simulink model "SP_Dynamic_17Okt_ExergyFlow"  (R2019b)
settings: Solver=FixedStepAuto  StartTime=0.0  StopTime=0  FixedStep=1/3600  RelTol=1e-3
model workspace (MAT data in the model file):
  AD : Simulink.Parameter (value not decoded)
  AG : Simulink.Parameter (value not decoded)
  AH : Simulink.Parameter (value not decoded)
  AV : Simulink.Parameter (value not decoded)
  AVP : Simulink.Parameter (value not decoded)
  BCHL : Simulink.Parameter (value not decoded)
  BCHV : Simulink.Parameter (value not decoded)
  BD : Simulink.Parameter (value not decoded)
  BG : Simulink.Parameter (value not decoded)
  BH : Simulink.Parameter (value not decoded)
  BVP : Simulink.Parameter (value not decoded)
  CD : Simulink.Parameter (value not decoded)
  CG : Simulink.Parameter (value not decoded)
  CH : Simulink.Parameter (value not decoded)
  CVP : Simulink.Parameter (value not decoded)
  XMW : Simulink.Parameter (value not decoded)
symbols that are objects in the model workspace (value not decoded): AD, AG, AH, AV, AVP, BD, BG, BH, BVP, CD, CG, CH, CVP, XMW
undefined symbols (not defined in the file or in its folder): magnitude, SETPT, XMEAS, XMV
libraries: mylib x165, dspindex x17
(part 6 of 10)

== system SP_Dynamic_17Okt_ExergyFlow/Reactor/Holdup of Components in Reactor/YP(3) ==
  FCM(3,7) : Inport
  CRXR(3) : Inport  Port=2
  FCM(3,8) : Inport  Port=3
  " " : Sum  Inputs=+-+
  Bus Selector : BusSelector  OutputSignals=CRXR(3)
  Bus Selector1 : BusSelector  OutputSignals=FCM(3;8)
  Bus Selector2 : BusSelector  OutputSignals=FCM(3;7)
  YP(3) : Integrator  InitialConditionSource=external
  "YY(3) " : Constant  Value=7.5700579737
  YY(3) : Outport  VectorParamsAs1DForOutWhenUnconnected=off
  wires:
  "YY(3) "/1 -> YP(3)/2
  CRXR(3)/1 -> Bus Selector/1
  FCM(3,8)/1 -> Bus Selector1/1
  FCM(3,7)/1 -> Bus Selector2/1
  " "/1 -> YP(3)/1
  YP(3)/1 -> YY(3)/1
  Bus Selector/1 -> " "/3  "<CRXR(3)>"
  Bus Selector1/1 -> " "/2  "<FCM(3;8)>"
  Bus Selector2/1 -> " "/1  "<FCM(3;7)>"

== system SP_Dynamic_17Okt_ExergyFlow/Reactor/Holdup of Components in Reactor/YP(4) ==
  FCM(4,7) : Inport
  CRXR(4) : Inport  Port=2
  FCM(4,8) : Inport  Port=3
  " " : Sum  Inputs=+-+
  Bus Selector : BusSelector  OutputSignals=CRXR(4)
  Bus Selector1 : BusSelector  OutputSignals=FCM(4;8)
  Bus Selector2 : BusSelector  OutputSignals=FCM(4;7)
  YP(4) : Integrator  InitialConditionSource=external
  YY(4) : Constant  Value=0.4230042431
  "YY(4) " : Outport  VectorParamsAs1DForOutWhenUnconnected=off
  wires:
  YY(4)/1 -> YP(4)/2
  CRXR(4)/1 -> Bus Selector/1
  FCM(4,8)/1 -> Bus Selector1/1
  FCM(4,7)/1 -> Bus Selector2/1
  " "/1 -> YP(4)/1
  YP(4)/1 -> "YY(4) "/1
  Bus Selector/1 -> " "/3  "<CRXR(4)>"
  Bus Selector1/1 -> " "/2  "<FCM(4;8)>"
  Bus Selector2/1 -> " "/1  "<FCM(4;7)>"

== system SP_Dynamic_17Okt_ExergyFlow/Reactor/Holdup of Components in Reactor/YP(5) ==
  FCM(5,7) : Inport
  CRXR(5) : Inport  Port=2
  FCM(5,8) : Inport  Port=3
  " " : Sum  Inputs=+-+
  Bus Selector : BusSelector  OutputSignals=CRXR(5)
  Bus Selector1 : BusSelector  OutputSignals=FCM(5;8)
  Bus Selector2 : BusSelector  OutputSignals=FCM(5;7)
  YP(5) : Integrator  InitialConditionSource=external
  YY(5) : Constant  Value=24.15513437
  "YY(5) " : Outport  VectorParamsAs1DForOutWhenUnconnected=off
  wires:
  YY(5)/1 -> YP(5)/2
  CRXR(5)/1 -> Bus Selector/1
  FCM(5,8)/1 -> Bus Selector1/1
  FCM(5,7)/1 -> Bus Selector2/1
  " "/1 -> YP(5)/1
  YP(5)/1 -> "YY(5) "/1
  Bus Selector/1 -> " "/3  "<CRXR(5)>"
  Bus Selector1/1 -> " "/2  "<FCM(5;8)>"
  Bus Selector2/1 -> " "/1  "<FCM(5;7)>"

== system SP_Dynamic_17Okt_ExergyFlow/Reactor/Holdup of Components in Reactor/YP(6) ==
  FCM(6,7) : Inport
  CRXR(6) : Inport  Port=2
  FCM(6,8) : Inport  Port=3
  " " : Sum  Inputs=+-+
  Bus Selector : BusSelector  OutputSignals=CRXR(6)
  Bus Selector1 : BusSelector  OutputSignals=FCM(6;8)
  Bus Selector2 : BusSelector  OutputSignals=FCM(6;7)
  YP(6) : Integrator  InitialConditionSource=external
  YY(6) : Constant  Value=2.942597645
  "YY(6) " : Outport  VectorParamsAs1DForOutWhenUnconnected=off
  wires:
  YY(6)/1 -> YP(6)/2
  CRXR(6)/1 -> Bus Selector/1
  FCM(6,8)/1 -> Bus Selector1/1
  FCM(6,7)/1 -> Bus Selector2/1
  " "/1 -> YP(6)/1
  YP(6)/1 -> "YY(6) "/1
  Bus Selector/1 -> " "/3  "<CRXR(6)>"
  Bus Selector1/1 -> " "/2  "<FCM(6;8)>"
  Bus Selector2/1 -> " "/1  "<FCM(6;7)>"

== system SP_Dynamic_17Okt_ExergyFlow/Reactor/Holdup of Components in Reactor/YP(7) ==
  FCM(7,7) : Inport
  CRXR(7) : Inport  Port=2
  FCM(7,8) : Inport  Port=3
  " " : Sum  Inputs=+-+
  Bus Selector : BusSelector  OutputSignals=CRXR(7)
  Bus Selector1 : BusSelector  OutputSignals=FCM(7;8)
  Bus Selector2 : BusSelector  OutputSignals=FCM(7;7)
  YP(7) : Integrator  InitialConditionSource=external
  YY(7) : Constant  Value=154.3770655
  "YY(7) " : Outport  VectorParamsAs1DForOutWhenUnconnected=off
  wires:
  YY(7)/1 -> YP(7)/2
  CRXR(7)/1 -> Bus Selector/1
  FCM(7,8)/1 -> Bus Selector1/1
  FCM(7,7)/1 -> Bus Selector2/1
  " "/1 -> YP(7)/1
  YP(7)/1 -> "YY(7) "/1
  Bus Selector/1 -> " "/3  "<CRXR(7)>"
  Bus Selector1/1 -> " "/2  "<FCM(7;8)>"
  Bus Selector2/1 -> " "/1  "<FCM(7;7)>"

== system SP_Dynamic_17Okt_ExergyFlow/Reactor/Holdup of Components in Reactor/YP(8) ==
  FCM(8,7) : Inport
  CRXR(8) : Inport  Port=2
  FCM(8,8) : Inport  Port=3
  " " : Sum  Inputs=+-+
  Bus Selector : BusSelector  OutputSignals=CRXR(8)
  Bus Selector1 : BusSelector  OutputSignals=FCM(8;8)
  Bus Selector2 : BusSelector  OutputSignals=FCM(8;7)
  YP(8) : Integrator  InitialConditionSource=external
  YY(8) : Constant  Value=159.1865960
  "YY(8) " : Outport  VectorParamsAs1DForOutWhenUnconnected=off
  wires:
  YY(8)/1 -> YP(8)/2
  CRXR(8)/1 -> Bus Selector/1
  FCM(8,8)/1 -> Bus Selector1/1
  FCM(8,7)/1 -> Bus Selector2/1
  " "/1 -> YP(8)/1
  YP(8)/1 -> "YY(8) "/1
  Bus Selector/1 -> " "/3  "<CRXR(8)>"
  Bus Selector1/1 -> " "/2  "<FCM(8;8)>"
  Bus Selector2/1 -> " "/1  "<FCM(8;7)>"

== system SP_Dynamic_17Okt_ExergyFlow/Reactor/Pressure of Reactor/Subsystem ==
  TKR : Inport
  VVR : Inport  Port=2
  UCVR : Inport  Port=3
  Bus Selector : BusSelector  OutputSignals=UCVR(1),UCVR(2),UCVR(3)
  PPR(1) Partial pressure of Component A mmHg : Product  Inputs=***/
  PPR(2) Partial pressure of Component B mmHg : Product  Inputs=***/
  PPR(3) Partial pressure of Component C mmHg : Product  Inputs=***/
  RG Universal Gas Constant ft³·mmHg/K·lb-mol : Constant  Value=998.9
  PPR(1) : Outport  VectorParamsAs1DForOutWhenUnconnected=off
  PPR(2) : Outport  Port=2  VectorParamsAs1DForOutWhenUnconnected=off
  PPR(3) : Outport  Port=3  VectorParamsAs1DForOutWhenUnconnected=off
  wires:
  Bus Selector/2 -> PPR(2) Partial pressure of Component B mmHg/1  "<UCVR(2)>"
  TKR/1 -> PPR(3) Partial pressure of Component C mmHg/3, PPR(2) Partial pressure of Component B mmHg/3, PPR(1) Partial pressure of Component A mmHg/3
  VVR/1 -> PPR(3) Partial pressure of Component C mmHg/4, PPR(2) Partial pressure of Component B mmHg/4, PPR(1) Partial pressure of Component A mmHg/4
  RG Universal Gas Constant ft³·mmHg/K·lb-mol/1 -> PPR(3) Partial pressure of Component C mmHg/2, PPR(1) Partial pressure of Component A mmHg/2, PPR(2) Partial pressure of Component B mmHg/2
  PPR(2) Partial pressure of Component B mmHg/1 -> PPR(2)/1  "PPR(2)"
  Bus Selector/1 -> PPR(1) Partial pressure of Component A mmHg/1  "<UCVR(1)>"
  Bus Selector/3 -> PPR(3) Partial pressure of Component C mmHg/1  "<UCVR(3)>"
  PPR(1) Partial pressure of Component A mmHg/1 -> PPR(1)/1  "PPR(1)"
  PPR(3) Partial pressure of Component C mmHg/1 -> PPR(3)/1  "PPR(3)"
  UCVR/1 -> Bus Selector/1

== system SP_Dynamic_17Okt_ExergyFlow/Reactor/Pressure of Reactor/VPR Vapour Pressure mmHg ==
  TCR : Inport
  AVP(I) Antoine Coefficient A ln(mmHg) : Constant  Value=AVP
  Add : Sum
  Add1 : Sum
  BVP(I) Antoine Coefficient B ln(mmHg)·°C : Constant  Value=BVP
  CVP(I) Antoine Coefficient C °C : Constant  Value=CVP
  Divide : Product  Inputs=*/
  Math Function : Math  SaturateOnIntegerOverflow=on
  VPR : Outport  VectorParamsAs1DForOutWhenUnconnected=off
  wires:
  BVP(I) Antoine Coefficient B ln(mmHg)·°C/1 -> Divide/1
  CVP(I) Antoine Coefficient C °C/1 -> Add/1
  AVP(I) Antoine Coefficient A ln(mmHg)/1 -> Add1/1
  Add/1 -> Divide/2
  Divide/1 -> Add1/2
  Add1/1 -> Math Function/1
  Math Function/1 -> VPR/1
  TCR/1 -> Add/2

== system SP_Dynamic_17Okt_ExergyFlow/Reactor/Reaction Rates/Component reaction rate lb-mol//h ==
  RR : Inport
  Bus Creator : BusCreator  Inputs=7
  Subsystem : Subsystem
  Subsystem1 : Subsystem
  Subsystem2 : Subsystem
  Subsystem3 : Subsystem
  Subsystem4 : Subsystem
  Subsystem5 : Subsystem
  Subsystem6 : Subsystem
  CRXR : Outport  VectorParamsAs1DForOutWhenUnconnected=off
  wires:
  RR/1 -> Subsystem4/1(RR), Subsystem6/1(RR), Subsystem5/1(RR), Subsystem3/1(RR), Subsystem1/1(RR), Subsystem/1(RR), Subsystem2/1(RR)
  Bus Creator/1 -> CRXR/1
  Subsystem/1(CRXR(1)) -> Bus Creator/1
  Subsystem1/1(CRXR(3)) -> Bus Creator/2
  Subsystem2/1(CRXR(4)) -> Bus Creator/3
  Subsystem3/1(CRXR(5)) -> Bus Creator/4
  Subsystem4/1(CRXR(6)) -> Bus Creator/5
  Subsystem5/1(CRXR(7)) -> Bus Creator/6
  Subsystem6/1(CRXR(8)) -> Bus Creator/7

== system SP_Dynamic_17Okt_ExergyFlow/Reactor/Reaction Rates/Reaction Heat MBtu//h ==
  RR : Inport
  Bus Selector : BusSelector  OutputSignals=RR(1),RR(2)
  HTR(1) Heat of Reaction 1 MBtu/lb-mol : Constant  Value=0.06899381054
  HTR(2) Heat of reaction 2 MBtu/lb-mol : Constant  Value=0.05
  Product : Product
  Product1 : Product
  RH Total reaction heat MBtu/h : Sum
  RH : Outport  VectorParamsAs1DForOutWhenUnconnected=off
  wires:
  HTR(2) Heat of reaction 2 MBtu/lb-mol/1 -> Product1/2
  Product/1 -> RH Total reaction heat MBtu/h/1
  Product1/1 -> RH Total reaction heat MBtu/h/2
  HTR(1) Heat of Reaction 1 MBtu/lb-mol/1 -> Product/2
  RH Total reaction heat MBtu/h/1 -> RH/1
  RR/1 -> Bus Selector/1
  Bus Selector/1 -> Product/1  "<RR(1)>"
  Bus Selector/2 -> Product1/1  "<RR(2)>"

== system SP_Dynamic_17Okt_ExergyFlow/Reactor/Reaction Rates/Reaction rates lb-mol//h ==
  TKR : Inport
  PPR : Inport  Port=2
  VVR : Inport  Port=3
  " Reaction rate of reaction 4 lb-mol/ft3·h    " : Subsystem
  Bus Creator : BusCreator  Inputs=4
  Product{,1..3} (4 alike) : Product
  Reaction rate of reaction 1 lb-mol/ft3·h : Subsystem
  Reaction rate of reaction 2 lb-mol/ft3·h : Subsystem
  "Reaction rate of reaction 3 lb-mol/ft3·h  " : Subsystem
  RR : Outport  VectorParamsAs1DForOutWhenUnconnected=off
  wires:
  TKR/1 -> Reaction rate of reaction 1 lb-mol/ft3·h/2(TKR), " Reaction rate of reaction 4 lb-mol/ft3·h    "/2(TKR), "Reaction rate of reaction 3 lb-mol/ft3·h  "/2(TKR), Reaction rate of reaction 2 lb-mol/ft3·h/2(TKR)
  PPR/1 -> Reaction rate of reaction 1 lb-mol/ft3·h/1(PPR), " Reaction rate of reaction 4 lb-mol/ft3·h    "/1(PPR), "Reaction rate of reaction 3 lb-mol/ft3·h  "/1(PPR), Reaction rate of reaction 2 lb-mol/ft3·h/1(PPR)
  Bus Creator/1 -> RR/1
  Reaction rate of reaction 1 lb-mol/ft3·h/1(RR(1)) -> Product/1  "RR(1)"
  VVR/1 -> Product/2, Product3/2, Product2/2, Product1/2
  Product/1 -> Bus Creator/1  "RR(1)"
  Reaction rate of reaction 2 lb-mol/ft3·h/1(RR(2)) -> Product1/1  "RR(2)"
  Product1/1 -> Bus Creator/2  "RR(2)"
  "Reaction rate of reaction 3 lb-mol/ft3·h  "/1(RR(3)) -> Product2/1  "RR(3)"
  Product2/1 -> Bus Creator/3  "RR(3)"
  " Reaction rate of reaction 4 lb-mol/ft3·h    "/1(RR(4)) -> Product3/1  "RR(4)"
  Product3/1 -> Bus Creator/4  "RR(4)"

== system SP_Dynamic_17Okt_ExergyFlow/Reactor/Reactor Heat exchanger/Position of Valve 10 % ==
  Bus Selector : BusSelector  OutputSignals=XMV(10)
  Bus Selector1 : BusSelector  OutputSignals=IDV(14)
  Control valve : mylib/Control valve  SystemSampleTime=-1  Latency=0  AutoFrameSizeCalculation=off
  Divide : Product  Inputs=*/
  Subtract : Sum  Inputs=+-
  VTAU(10) : Constant  Value=5/3600
  YP(48) : Integrator  InitialConditionSource=external
  YY(48) : Constant  Value=41.10581288
  "YY(48) " : Outport  PortDimensions=1  VectorParamsAs1DForOutWhenUnconnected=off
  wires:
  YP(48)/1 -> Subtract/2, "YY(48) "/1  "VPOS(10)"
  Subtract/1 -> Divide/1
  Control valve/1 -> Subtract/1
  VTAU(10)/1 -> Divide/2
  Divide/1 -> YP(48)/1
  YY(48)/1 -> YP(48)/2
  [XMV] -> Bus Selector/1
  Bus Selector/1 -> Control valve/1  "<XMV(10)>"
  [IDV] -> Bus Selector1/1
  Bus Selector1/1 -> Control valve/2  "<IDV(14)>"

== system SP_Dynamic_17Okt_ExergyFlow/Reactor/Reactor Heat exchanger/Position of Valve 12 % ==
  Bus Selector : BusSelector  OutputSignals=XMV(12)
  Control valve : Subsystem
  Divide : Product  Inputs=*/
  Subtract : Sum  Inputs=+-
  VTAU(12) : Constant  Value=5/3600
  YP(50) : Integrator  InitialConditionSource=external
  YY(50) : Constant  Value=50
  "YY(50) " : Outport  PortDimensions=1  VectorParamsAs1DForOutWhenUnconnected=off
  wires:
  YP(50)/1 -> Subtract/2, "YY(50) "/1  "VPOS(12)"
  Subtract/1 -> Divide/1
  Control valve/1(VCV(12)) -> Subtract/1
  VTAU(12)/1 -> Divide/2
  Divide/1 -> YP(50)/1
  YY(50)/1 -> YP(50)/2
  [XMV] -> Bus Selector/1
  Bus Selector/1 -> Control valve/1(XMV(12))  "<XMV(12)>"

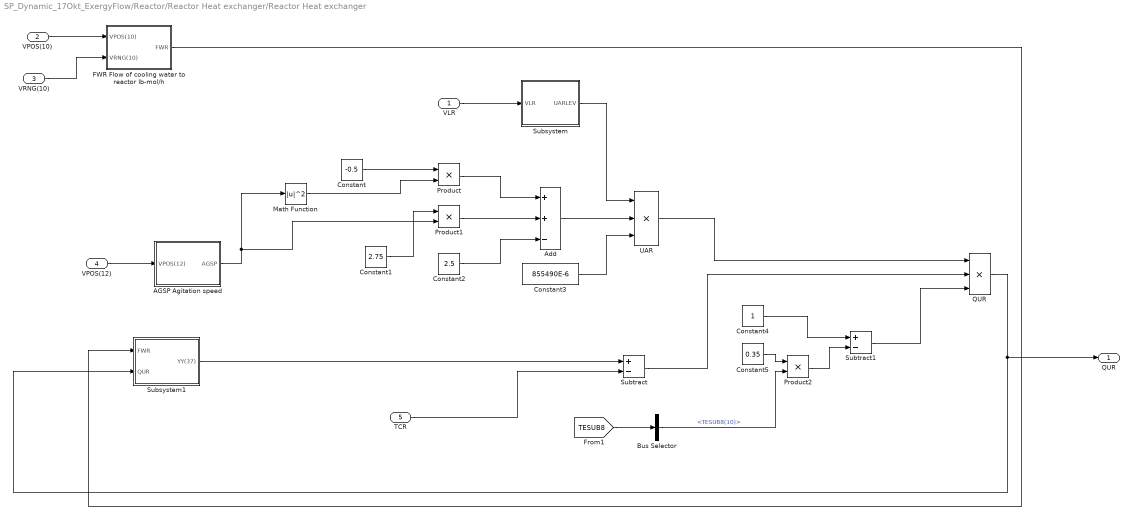
== system SP_Dynamic_17Okt_ExergyFlow/Reactor/Reactor Heat exchanger/Reactor Heat exchanger ==
  VLR : Inport
  VPOS(10) : Inport  Port=2
  VRNG(10) : Inport  Port=3
  VPOS(12) : Inport  Port=4
  TCR : Inport  Port=5
  AGSP Agitation speed : Subsystem
  Add : Sum  Inputs=++-
  Bus Selector : BusSelector  OutputSignals=TESUB8(10)
  Constant : Constant  Value=-0.5
  Constant1 : Constant  Value=2.75
  Constant2 : Constant  Value=2.5
  Constant3 : Constant  Value=855490E-6
  Constant4 : Constant
  Constant5 : Constant  Value=0.35
  FWR Flow of cooling water to reactor lb-mol/h : Subsystem
  Math Function : Math  Operator=magnitude^2  SaturateOnIntegerOverflow=on
  Product : Product
  Product1 : Product
  Product2 : Product
  QUR : Product  Inputs=3
  Subsystem : Subsystem
  Subsystem1 : Subsystem
  Subtract : Sum  Inputs=+-
  Subtract1 : Sum  Inputs=+-
  UAR : Product  Inputs=3
  "QUR " : Outport  PortDimensions=1  VectorParamsAs1DForOutWhenUnconnected=off
  wires:
  VRNG(10)/1 -> FWR Flow of cooling water to reactor lb-mol/h/2(VRNG(10))
  VLR/1 -> Subsystem/1(VLR)
  VPOS(10)/1 -> FWR Flow of cooling water to reactor lb-mol/h/1(VPOS(10))
  VPOS(12)/1 -> AGSP Agitation speed/1(VPOS(12))
  AGSP Agitation speed/1(AGSP) -> Product1/2, Math Function/1
  Constant/1 -> Product/1
  Math Function/1 -> Product/2
  Constant1/1 -> Product1/1
  Product/1 -> Add/1
  Product1/1 -> Add/2
  Constant2/1 -> Add/3
  Subsystem/1("UARLEV ") -> UAR/1
  Add/1 -> UAR/2
  Constant3/1 -> UAR/3
  Subsystem1/1("YY(37) ") -> Subtract/1
  TCR/1 -> Subtract/2
  UAR/1 -> QUR/1
  Subtract/1 -> QUR/2
  Constant5/1 -> Product2/1
  Bus Selector/1 -> Product2/2  "<TESUB8(10)>"
  Constant4/1 -> Subtract1/1
  Product2/1 -> Subtract1/2
  Subtract1/1 -> QUR/3
  FWR Flow of cooling water to reactor lb-mol/h/1(FWR) -> Subsystem1/1(FWR)
  QUR/1 -> "QUR "/1, Subsystem1/2(QUR)
  [TESUB8] -> Bus Selector/1

== system SP_Dynamic_17Okt_ExergyFlow/Reactor/Stream 8/HST(8) Molar Enthalpy of Stream 8 MBtu//lb-mol ==
  ITY : Inport
  T : Inport  Port=2
  XST(I,I) : Inport  Port=3
  "Enthalpy of Stream " : mylib/Enthalpy of Stream   SystemSampleTime=-1  Latency=0  AutoFrameSizeCalculation=off
  "H " : Outport  VectorParamsAs1DForOutWhenUnconnected=off
  wires:
  ITY/1 -> "Enthalpy of Stream "/1
  T/1 -> "Enthalpy of Stream "/2
  XST(I,I)/1 -> "Enthalpy of Stream "/3
  "Enthalpy of Stream "/1 -> "H "/1

== system SP_Dynamic_17Okt_ExergyFlow/Reactor/Stream 8/Subsystem ==
  Abs : Abs
  Bus Selector : BusSelector  OutputSignals=TESUB8(12)
  Constant : Constant  Value=0.0
  Constant1 : Constant  Value=4574.21
  Constant2 : Constant
  Constant3 : Constant  Value=0.25
  DLP : Sum  Inputs=+-
  DLP Pressure drop between separator and reactor : Merge
  FLMS : Product  Inputs=3
  If : If  IfExpression=u1 < 0
  If Action Subsystem : Subsystem  TreatAsAtomicUnit=on
  If Action Subsystem1 : Subsystem  TreatAsAtomicUnit=on
  Product : Product
  Sqrt : Sqrt  SaturateOnIntegerOverflow=on
  Subtract : Sum  Inputs=+-
  "FLMS " : Outport  VectorParamsAs1DForOutWhenUnconnected=off
  wires:
  [PTS] -> DLP/2
  If Action Subsystem/1(Out1) -> DLP Pressure drop between separator and reactor/1
  Constant2/1 -> Subtract/1
  DLP/1 -> If/1, If Action Subsystem1/1(In1)
  DLP Pressure drop between separator and reactor/1 -> Abs/1
  If Action Subsystem1/1(Out1) -> DLP Pressure drop between separator and reactor/2
  If/1 -> If Action Subsystem/Action
  Sqrt/1 -> FLMS/2
  [PTR] -> DLP/1
  Abs/1 -> Sqrt/1
  Constant3/1 -> Product/1
  Constant1/1 -> FLMS/1
  [TESUB8] -> Bus Selector/1
  Subtract/1 -> FLMS/3
  Bus Selector/1 -> Product/2  "<TESUB8(12)>"
  If/2 -> If Action Subsystem1/Action
  Product/1 -> Subtract/2
  Constant/1 -> If Action Subsystem/1(In1)
  FLMS/1 -> "FLMS "/1

== system SP_Dynamic_17Okt_ExergyFlow/Reactor/Stream 8/XMWS(8) Molecular weight of Stream 8 lb//lb-mol ==
  XST(I,8) : Inport
  Product : Product
  Sum of Elements : Sum  Inputs=+
  "XMW(I) Molecular weight of components lb/lb-mol " : Constant  Value=[2;25.4;28;32;46;48;62;76]
  XMWS(8) : Outport  VectorParamsAs1DForOutWhenUnconnected=off
  wires:
  Sum of Elements/1 -> XMWS(8)/1
  Product/1 -> Sum of Elements/1
  XST(I,8)/1 -> Product/1
  "XMW(I) Molecular weight of components lb/lb-mol "/1 -> Product/2

== system SP_Dynamic_17Okt_ExergyFlow/Reactor/Volume of Reactor/DLR Molar Density of Liquids in Reactor lb-mol//ft³     ==
  XLR : Inport
  TCR : Inport  Port=2
  "DLR Molar Density of Liquids in Reactor lb-mol/ft³ " : Subsystem
  "DLR " : Outport  VectorParamsAs1DForOutWhenUnconnected=off
  wires:
  "DLR Molar Density of Liquids in Reactor lb-mol/ft³ "/1("R ") -> "DLR "/1
  TCR/1 -> "DLR Molar Density of Liquids in Reactor lb-mol/ft³ "/2(T)
  XLR/1 -> "DLR Molar Density of Liquids in Reactor lb-mol/ft³ "/1(X)

== system SP_Dynamic_17Okt_ExergyFlow/Separator/Holdup of Components in Separator/Holdup of Liquid Components in Separator ==
  YY(10:17) : Inport
  Bus Creator : BusCreator  Inputs=8
  Bus Selector : BusSelector  OutputSignals=YY(13),YY(14),YY(15),YY(16),YY(17)
  UCLS(1) Holdup of Component A (Liquid) in Separator lb-mol : Constant  Value=0
  UCLS(2) Holdup of Component B (Liquid) in Separator lb-mol : Constant  Value=0
  UCLS(4) Holdup of Component D (Liquid) in Separator lb-mol : Gain
  UCLS(5) Holdup of Component E (Liquid) in Separator lb-mol : Gain
  UCLS(6) Holdup of Component F (Liquid) in Separator lb-mol : Gain
  UCLS(7) Holdup of Component G (Liquid) in Separator lb-mol : Gain
  UCLS(8) Holdup of Component H (Liquid) in Separator lb-mol : Gain
  UCLS3) Holdup of Component C (Liquid) in Separator lb-mol : Constant  Value=0
  UCLS : Outport  VectorParamsAs1DForOutWhenUnconnected=off
  wires:
  UCLS(2) Holdup of Component B (Liquid) in Separator lb-mol/1 -> Bus Creator/2  "UCLS(2)"
  UCLS(8) Holdup of Component H (Liquid) in Separator lb-mol/1 -> Bus Creator/8  "UCLS(8)"
  UCLS(1) Holdup of Component A (Liquid) in Separator lb-mol/1 -> Bus Creator/1  "UCLS(1)"
  UCLS(5) Holdup of Component E (Liquid) in Separator lb-mol/1 -> Bus Creator/5  "UCLS(5)"
  UCLS(4) Holdup of Component D (Liquid) in Separator lb-mol/1 -> Bus Creator/4  "UCLS(4)"
  UCLS3) Holdup of Component C (Liquid) in Separator lb-mol/1 -> Bus Creator/3  "UCLS(3)"
  UCLS(6) Holdup of Component F (Liquid) in Separator lb-mol/1 -> Bus Creator/6  "UCLS(6)"
  UCLS(7) Holdup of Component G (Liquid) in Separator lb-mol/1 -> Bus Creator/7  "UCLS(7)"
  YY(10:17)/1 -> Bus Selector/1
  Bus Creator/1 -> UCLS/1
  Bus Selector/1 -> UCLS(4) Holdup of Component D (Liquid) in Separator lb-mol/1  "<YY(13)>"
  Bus Selector/2 -> UCLS(5) Holdup of Component E (Liquid) in Separator lb-mol/1  "<YY(14)>"
  Bus Selector/3 -> UCLS(6) Holdup of Component F (Liquid) in Separator lb-mol/1  "<YY(15)>"
  Bus Selector/4 -> UCLS(7) Holdup of Component G (Liquid) in Separator lb-mol/1  "<YY(16)>"
  Bus Selector/5 -> UCLS(8) Holdup of Component H (Liquid) in Separator lb-mol/1  "<YY(17)>"

== system SP_Dynamic_17Okt_ExergyFlow/Separator/Holdup of Components in Separator/Holdup of Vapour Components in Separator ==
  YY(10:17) : Inport
  Bus Creator : BusCreator  Inputs=3
  Bus Selector : BusSelector  OutputSignals=YY(10),YY(11),YY(12)
  UCVS(1) Holdup of Component A (Vapour) in Separator lb-mol : Gain
  UCVS(2) Holdup of Component B (Vapour) in Separator lb-mol : Gain
  UCVS(3) Holdup of Component C (Vapour) in Separator lb-mol : Gain
  UCVS : Outport  VectorParamsAs1DForOutWhenUnconnected=off
  wires:
  UCVS(1) Holdup of Component A (Vapour) in Separator lb-mol/1 -> Bus Creator/1  "UCVS(1)"
  Bus Selector/3 -> UCVS(3) Holdup of Component C (Vapour) in Separator lb-mol/1  "<YY(12)>"
  UCVS(2) Holdup of Component B (Vapour) in Separator lb-mol/1 -> Bus Creator/2  "UCVS(2)"
  UCVS(3) Holdup of Component C (Vapour) in Separator lb-mol/1 -> Bus Creator/3  "UCVS(3)"
  Bus Creator/1 -> UCVS/1
  YY(10:17)/1 -> Bus Selector/1
  Bus Selector/1 -> UCVS(1) Holdup of Component A (Vapour) in Separator lb-mol/1  "<YY(10)>"
  Bus Selector/2 -> UCVS(2) Holdup of Component B (Vapour) in Separator lb-mol/1  "<YY(11)>"

== system SP_Dynamic_17Okt_ExergyFlow/Separator/Holdup of Components in Separator/Liquid Component Fraction in Separator ==
  UTLS : Inport
  UCLS : Inport  Port=2
  Bus Creator : BusCreator  Inputs=8
  Bus Selector : BusSelector  OutputSignals=UCLS(1),UCLS(2),UCLS(3),UCLS(4),UCLS(5),UCLS(6),UCLS(7),UCLS(8)
  Display : Display
  Display1 : Display
  Display2 : Display
  XLS(1) : Product  Inputs=*/
  XLS(2) : Product  Inputs=*/
  XLS(3) : Product  Inputs=*/
  XLS(4) : Product  Inputs=*/
  XLS(5) : Product  Inputs=*/
  XLS(6) : Product  Inputs=*/
  XLS(7) : Product  Inputs=*/
  XLS(8) : Product  Inputs=*/
  XLS : Outport  VectorParamsAs1DForOutWhenUnconnected=off
  wires:
  Bus Selector/1 -> XLS(1)/1  "<UCLS(1)>"
  XLS(2)/1 -> Bus Creator/2  "XLS(2)"
  Bus Selector/7 -> XLS(7)/1  "<UCLS(7)>"
  XLS(3)/1 -> Bus Creator/3  "XLS(3)"
  Bus Selector/8 -> XLS(8)/1  "<UCLS(8)>"
  Bus Selector/3 -> XLS(3)/1  "<UCLS(3)>"
  XLS(7)/1 -> Bus Creator/7  "XLS(7)"
  XLS(1)/1 -> Bus Creator/1  "XLS(1)"
  Bus Selector/2 -> XLS(2)/1  "<UCLS(2)>"
  Bus Selector/5 -> XLS(5)/1  "<UCLS(5)>"
  Bus Selector/4 -> XLS(4)/1  "<UCLS(4)>"
  XLS(6)/1 -> Bus Creator/6  "XLS(6)"
  XLS(4)/1 -> Bus Creator/4  "XLS(4)"
  XLS(5)/1 -> Bus Creator/5  "XLS(5)"
  XLS(8)/1 -> Bus Creator/8  "XLS(8)"
  Bus Selector/6 -> XLS(6)/1  "<UCLS(6)>"
  Bus Creator/1 -> Display/1, XLS/1
  UTLS/1 -> XLS(8)/2, XLS(7)/2, XLS(6)/2, XLS(5)/2, XLS(4)/2, XLS(3)/2, XLS(2)/2, Display2/1, XLS(1)/2
  UCLS/1 -> Display1/1, Bus Selector/1

== system SP_Dynamic_17Okt_ExergyFlow/Separator/Holdup of Components in Separator/YP(10) ==
  FCM(1,8) : Inport
  FCM(1,9) : Inport  Port=2
  FCM(1,10) : Inport  Port=3
  FCM(1,11) : Inport  Port=4
  " " : Sum  Inputs=+---
  YP(10) : Integrator  InitialConditionSource=external
  "YY(10) " : Constant  Value=63.75581199
  YY(10) : Outport  VectorParamsAs1DForOutWhenUnconnected=off
  wires:
  "YY(10) "/1 -> YP(10)/2
  FCM(1,10)/1 -> " "/3
  FCM(1,9)/1 -> " "/2
  FCM(1,8)/1 -> " "/1
  " "/1 -> YP(10)/1
  YP(10)/1 -> YY(10)/1
  FCM(1,11)/1 -> " "/4

== system SP_Dynamic_17Okt_ExergyFlow/Separator/Holdup of Components in Separator/YP(11) ==
  FCM(2,8) : Inport
  FCM(2,9) : Inport  Port=2
  FCM(2,10) : Inport  Port=3
  FCM(2,11) : Inport  Port=4
  " " : Sum  Inputs=+---
  YP(11) : Integrator  InitialConditionSource=external
  "YY(11) " : Constant  Value=26.74026066
  YY(11) : Outport  VectorParamsAs1DForOutWhenUnconnected=off
  wires:
  YP(11)/1 -> YY(11)/1
  FCM(2,8)/1 -> " "/1
  FCM(2,9)/1 -> " "/2
  FCM(2,10)/1 -> " "/3
  FCM(2,11)/1 -> " "/4
  "YY(11) "/1 -> YP(11)/2
  " "/1 -> YP(11)/1

== system SP_Dynamic_17Okt_ExergyFlow/Separator/Holdup of Components in Separator/YP(12) ==
  FCM(3,8) : Inport
  FCM(3,9) : Inport  Port=2
  FCM(3,10) : Inport  Port=3
  FCM(3,11) : Inport  Port=4
  " " : Sum  Inputs=+---
  YP(12) : Integrator  InitialConditionSource=external
  "YY(12) " : Constant  Value=46.38532432
  YY(12) : Outport  VectorParamsAs1DForOutWhenUnconnected=off
  wires:
  YP(12)/1 -> YY(12)/1
  FCM(3,8)/1 -> " "/1
  FCM(3,9)/1 -> " "/2
  FCM(3,10)/1 -> " "/3
  FCM(3,11)/1 -> " "/4
  " "/1 -> YP(12)/1
  "YY(12) "/1 -> YP(12)/2

== system SP_Dynamic_17Okt_ExergyFlow/Separator/Holdup of Components in Separator/YP(13) ==
  FCM(4,8) : Inport
  FCM(4,9) : Inport  Port=2
  FCM(4,10) : Inport  Port=3
  FCM(4,11) : Inport  Port=4
  " " : Sum  Inputs=+---
  YP(13) : Integrator  InitialConditionSource=external
  YY(13) : Constant  Value=0.2464521543
  "YY(13) " : Outport  VectorParamsAs1DForOutWhenUnconnected=off
  wires:
  YP(13)/1 -> "YY(13) "/1
  FCM(4,8)/1 -> " "/1
  FCM(4,9)/1 -> " "/2
  FCM(4,10)/1 -> " "/3
  FCM(4,11)/1 -> " "/4
  " "/1 -> YP(13)/1
  YY(13)/1 -> YP(13)/2

== system SP_Dynamic_17Okt_ExergyFlow/Separator/Holdup of Components in Separator/YP(14) ==
  FCM(5,8) : Inport
  FCM(5,9) : Inport  Port=2
  FCM(5,10) : Inport  Port=3
  FCM(5,11) : Inport  Port=4
  " " : Sum  Inputs=+---
  YP(14) : Integrator  InitialConditionSource=external
  YY(14) : Constant  Value=15.20484404
  "YY(14) " : Outport  VectorParamsAs1DForOutWhenUnconnected=off
  wires:
  YP(14)/1 -> "YY(14) "/1
  FCM(5,8)/1 -> " "/1
  FCM(5,9)/1 -> " "/2
  FCM(5,10)/1 -> " "/3
  FCM(5,11)/1 -> " "/4
  " "/1 -> YP(14)/1
  YY(14)/1 -> YP(14)/2

== system SP_Dynamic_17Okt_ExergyFlow/Separator/Holdup of Components in Separator/YP(15) ==
  FCM(6,8) : Inport
  FCM(6,9) : Inport  Port=2
  FCM(6,10) : Inport  Port=3
  FCM(6,11) : Inport  Port=4
  " " : Sum  Inputs=+---
  YP(15) : Integrator  InitialConditionSource=external
  YY(15) : Constant  Value=1.852266172
  "YY(15) " : Outport  VectorParamsAs1DForOutWhenUnconnected=off
  wires:
  YP(15)/1 -> "YY(15) "/1
  FCM(6,8)/1 -> " "/1
  FCM(6,9)/1 -> " "/2
  FCM(6,10)/1 -> " "/3
  FCM(6,11)/1 -> " "/4
  " "/1 -> YP(15)/1
  YY(15)/1 -> YP(15)/2

== system SP_Dynamic_17Okt_ExergyFlow/Separator/Holdup of Components in Separator/YP(16) ==
  FCM(7,8) : Inport
  FCM(7,9) : Inport  Port=2
  FCM(7,10) : Inport  Port=3
  FCM(7,11) : Inport  Port=4
  " " : Sum  Inputs=+---
  YP(16) : Integrator  InitialConditionSource=external
  YY(16) : Constant  Value=52.44639459
  "YY(16) " : Outport  VectorParamsAs1DForOutWhenUnconnected=off
  wires:
  YP(16)/1 -> "YY(16) "/1
  FCM(7,8)/1 -> " "/1
  FCM(7,9)/1 -> " "/2
  FCM(7,10)/1 -> " "/3
  FCM(7,11)/1 -> " "/4
  " "/1 -> YP(16)/1
  YY(16)/1 -> YP(16)/2

== system SP_Dynamic_17Okt_ExergyFlow/Separator/Holdup of Components in Separator/YP(17) ==
  FCM(8,8) : Inport
  FCM(8,9) : Inport  Port=2
  FCM(8,10) : Inport  Port=3
  FCM(8,11) : Inport  Port=4
  " " : Sum  Inputs=+---
  YP(17) : Integrator  InitialConditionSource=external
  YY(17) : Constant  Value=41.20394008
  "YY(17) " : Outport  VectorParamsAs1DForOutWhenUnconnected=off
  wires:
  YP(17)/1 -> "YY(17) "/1
  FCM(8,8)/1 -> " "/1
  FCM(8,9)/1 -> " "/2
  FCM(8,10)/1 -> " "/3
  " "/1 -> YP(17)/1
  YY(17)/1 -> YP(17)/2
  FCM(8,11)/1 -> " "/4

== system SP_Dynamic_17Okt_ExergyFlow/Separator/Pressure of Separator/Subsystem ==
  TCS : Inport
  VVS : Inport  Port=2
  UCVS : Inport  Port=3
  Bus Selector : BusSelector  OutputSignals=UCVS(1),UCVS(2),UCVS(3)
  PPS(1) Partial pressure of Component A mmHg : Product  Inputs=***/
  PPS(2) Partial pressure of Component B mmHg : Product  Inputs=***/
  PPS(3) Partial pressure of Component C mmHg : Product  Inputs=***/
  RG Universal Gas Constant ft³·mmHg/K·lb-mol : Constant  Value=998.9
  TKS Temperature in Separator K : Sum
  To Convert °C to K : Constant  Value=273.15
  PPS(1) : Outport  VectorParamsAs1DForOutWhenUnconnected=off
  PPS(2) : Outport  Port=2  VectorParamsAs1DForOutWhenUnconnected=off
  PPS(3) : Outport  Port=3  VectorParamsAs1DForOutWhenUnconnected=off
  wires:
  Bus Selector/3 -> PPS(3) Partial pressure of Component C mmHg/1  "<UCVS(3)>"
  RG Universal Gas Constant ft³·mmHg/K·lb-mol/1 -> PPS(3) Partial pressure of Component C mmHg/2, PPS(1) Partial pressure of Component A mmHg/2, PPS(2) Partial pressure of Component B mmHg/2
  UCVS/1 -> Bus Selector/1
  Bus Selector/1 -> PPS(1) Partial pressure of Component A mmHg/1  "<UCVS(1)>"
  Bus Selector/2 -> PPS(2) Partial pressure of Component B mmHg/1  "<UCVS(2)>"
  VVS/1 -> PPS(3) Partial pressure of Component C mmHg/4, PPS(2) Partial pressure of Component B mmHg/4, PPS(1) Partial pressure of Component A mmHg/4
  PPS(3) Partial pressure of Component C mmHg/1 -> PPS(3)/1
  To Convert °C to K/1 -> TKS Temperature in Separator K/2
  PPS(1) Partial pressure of Component A mmHg/1 -> PPS(1)/1
  TKS Temperature in Separator K/1 -> PPS(3) Partial pressure of Component C mmHg/3, PPS(2) Partial pressure of Component B mmHg/3, PPS(1) Partial pressure of Component A mmHg/3
  PPS(2) Partial pressure of Component B mmHg/1 -> PPS(2)/1
  TCS/1 -> TKS Temperature in Separator K/1

== system SP_Dynamic_17Okt_ExergyFlow/Separator/Pressure of Separator/VPR Vapour Pressure mmHg ==
  TCS : Inport
  AVP(I) Antoine Coefficient A ln(mmHg) : Constant  Value=AVP
  Add : Sum
  Add1 : Sum
  BVP(I) Antoine Coefficient B ln(mmHg)·°C : Constant  Value=BVP
  CVP(I) Antoine Coefficient C °C : Constant  Value=CVP
  Divide : Product  Inputs=*/
  Math Function : Math  SaturateOnIntegerOverflow=on
  VPR : Outport  VectorParamsAs1DForOutWhenUnconnected=off
  wires:
  BVP(I) Antoine Coefficient B ln(mmHg)·°C/1 -> Divide/1
  CVP(I) Antoine Coefficient C °C/1 -> Add/1
  AVP(I) Antoine Coefficient A ln(mmHg)/1 -> Add1/1
  Add/1 -> Divide/2
  Divide/1 -> Add1/2
  Add1/1 -> Math Function/1
  Math Function/1 -> VPR/1
  TCS/1 -> Add/2

== system SP_Dynamic_17Okt_ExergyFlow/Separator/Stream 10/HST(10) Molar Enthalpy of Stream 10 MBtu//lb-mol ==
  ITY : Inport
  T : Inport  Port=2
  XST(I,I) : Inport  Port=3
  "Enthalpy of Stream " : mylib/Enthalpy of Stream   SystemSampleTime=-1  Latency=0  AutoFrameSizeCalculation=off
  "H " : Outport  VectorParamsAs1DForOutWhenUnconnected=off
  wires:
  ITY/1 -> "Enthalpy of Stream "/1
  T/1 -> "Enthalpy of Stream "/2
  XST(I,I)/1 -> "Enthalpy of Stream "/3
  "Enthalpy of Stream "/1 -> "H "/1

== system SP_Dynamic_17Okt_ExergyFlow/Separator/Stream 10/Subsystem ==
  VPOS(6) : Inport  PortDimensions=1
  Abs : Abs
  Constant : Constant  Value=0.0
  Constant1 : Constant  Value=0.151169
  Constant2 : Constant  Value=760
  DLP : Sum  Inputs=+-
  DLP Pressure drop between separator and environment : Merge
  FLMS : Product  Inputs=3
  If : If  IfExpression=u1 < 0
  If Action Subsystem : Subsystem  TreatAsAtomicUnit=on
  If Action Subsystem1 : Subsystem  TreatAsAtomicUnit=on
  Sqrt : Sqrt  SaturateOnIntegerOverflow=on
  Out1 : Outport  VectorParamsAs1DForOutWhenUnconnected=off
  wires:
  Constant2/1 -> DLP/2
  Constant1/1 -> FLMS/2
  Abs/1 -> Sqrt/1
  DLP Pressure drop between separator and environment/1 -> Abs/1
  [PTS] -> DLP/1
  If Action Subsystem/1(Out1) -> DLP Pressure drop between separator and environment/1
  Constant/1 -> If Action Subsystem/1(In1)
  Sqrt/1 -> FLMS/3
  If Action Subsystem1/1(Out1) -> DLP Pressure drop between separator and environment/2
  If/2 -> If Action Subsystem1/Action
  DLP/1 -> If Action Subsystem1/1(In1), If/1
  VPOS(6)/1 -> FLMS/1
  If/1 -> If Action Subsystem/Action
  FLMS/1 -> Out1/1

== system SP_Dynamic_17Okt_ExergyFlow/Separator/Stream 10/XMWS(10) Molecular weight of Stream 10 lb//lb-mol ==
  XST(I,10) : Inport
  Constant : Constant  Value=XMW
  Product : Product
  Sum of Elements : Sum  Inputs=+
  XMWS(10) : Outport  VectorParamsAs1DForOutWhenUnconnected=off
  wires:
  Sum of Elements/1 -> XMWS(10)/1
  Product/1 -> Sum of Elements/1
  XST(I,10)/1 -> Product/1
  Constant/1 -> Product/2

== system SP_Dynamic_17Okt_ExergyFlow/Separator/Stream 11/HST(10) Molar Enthalpy of Stream 10 MBtu//lb-mol ==
  ITY : Inport
  T : Inport  Port=2
  XST(I,I) : Inport  Port=3
  "Enthalpy of Stream " : mylib/Enthalpy of Stream   SystemSampleTime=-1  Latency=0  AutoFrameSizeCalculation=off
  "H " : Outport  VectorParamsAs1DForOutWhenUnconnected=off
  wires:
  ITY/1 -> "Enthalpy of Stream "/1
  T/1 -> "Enthalpy of Stream "/2
  XST(I,I)/1 -> "Enthalpy of Stream "/3
  "Enthalpy of Stream "/1 -> "H "/1

== system SP_Dynamic_17Okt_ExergyFlow/Separator/Stream 9/HST(9) Molar Enthalpy of Stream 9 MBtu//lb-mol ==
  ITY : Inport
  T : Inport  Port=2
  XST(I,I) : Inport  Port=3
  "Enthalpy of Stream " : mylib/Enthalpy of Stream   SystemSampleTime=-1  Latency=0  AutoFrameSizeCalculation=off
  "H " : Outport  PortDimensions=1  VectorParamsAs1DForOutWhenUnconnected=off
  wires:
  ITY/1 -> "Enthalpy of Stream "/1
  T/1 -> "Enthalpy of Stream "/2
  XST(I,I)/1 -> "Enthalpy of Stream "/3
  "Enthalpy of Stream "/1 -> "H "/1

== system SP_Dynamic_17Okt_ExergyFlow/Separator/Stream 9/Subsystem ==
  VPOS(5) : Inport
  Abs : Abs
  Constant1 : Constant  Value=53.349
  Constant2 : Constant  Value=1E-3
  FLMS : Product  Inputs=3
  "FLMS  " : Merge
  If Action Subsystem2 : Subsystem  TreatAsAtomicUnit=on
  If Action Subsystem3 : Subsystem  TreatAsAtomicUnit=on
  If1 : If  IfExpression=u1 < 1E-3
  Pressure drop : Subsystem
  Sqrt : Sqrt  SaturateOnIntegerOverflow=on
  Subtract : Sum  Inputs=+-
  Out1 : Outport  VectorParamsAs1DForOutWhenUnconnected=off
  wires:
  FLMS/1 -> Subtract/2
  If1/1 -> If Action Subsystem2/Action
  [FLMS] -> Subtract/1
  Subtract/1 -> If Action Subsystem3/1(In1), If1/1
  If Action Subsystem3/1(Out1) -> "FLMS  "/2
  Abs/1 -> Sqrt/1
  Constant1/1 -> FLMS/2
  Sqrt/1 -> FLMS/3
  If1/2 -> If Action Subsystem3/Action
  Constant2/1 -> If Action Subsystem2/1(In1)
  VPOS(5)/1 -> FLMS/1
  If Action Subsystem2/1(Out1) -> "FLMS  "/1
  "FLMS  "/1 -> Out1/1
  Pressure drop/1(Out1) -> Abs/1

== system SP_Dynamic_17Okt_ExergyFlow/Separator/Stream 9/XMWS(9) Molecular weight of Stream 9 lb//lb-mol ==
  XST(I,9) : Inport
  Product : Product
  Sum of Elements : Sum  Inputs=+
  "XMW(I) Molecular weight of components lb/lb-mol " : Constant  Value=[2;25.4;28;32;46;48;62;76]
  XMWS(9) : Outport  VectorParamsAs1DForOutWhenUnconnected=off
  wires:
  Sum of Elements/1 -> XMWS(9)/1
  Product/1 -> Sum of Elements/1
  XST(I,9)/1 -> Product/1
  "XMW(I) Molecular weight of components lb/lb-mol "/1 -> Product/2

== system SP_Dynamic_17Okt_ExergyFlow/Separator/Volume of Separator/DLS Molar Density of Liquids in Reactor lb-mol//ft³     ==
  XLS : Inport
  TCS : Inport  Port=2
  "DLS Molar Density of Liquids in Separator lb-mol/ft³ " : Subsystem
  "DLS " : Outport  VectorParamsAs1DForOutWhenUnconnected=off
  wires:
  "DLS Molar Density of Liquids in Separator lb-mol/ft³ "/1("R ") -> "DLS "/1
  TCS/1 -> "DLS Molar Density of Liquids in Separator lb-mol/ft³ "/2(T)
  XLS/1 -> "DLS Molar Density of Liquids in Separator lb-mol/ft³ "/1(X)

== system SP_Dynamic_17Okt_ExergyFlow/Stripper/Heat transfer of stripper/If Action Subsystem ==
  In1 : Inport
  Action Port : ActionPort  ActionPortLabel=if(u1 < 100)
  Out1 : Outport  VectorParamsAs1DForOutWhenUnconnected=off
  wires:
  In1/1 -> Out1/1

== system SP_Dynamic_17Okt_ExergyFlow/Stripper/Heat transfer of stripper/If Action Subsystem1 ==
  In1 : Inport
  Action Port : ActionPort  ActionPortLabel=else
  Out1 : Outport  VectorParamsAs1DForOutWhenUnconnected=off
  wires:
  In1/1 -> Out1/1

== system SP_Dynamic_17Okt_ExergyFlow/Stripper/Holdup of Components in Stripper/Holsup of Liquid Components in Stripper ==
  YY(19:26) : Inport
  Bus Creator : BusCreator  Inputs=8
  Bus Selector : BusSelector  OutputSignals=YY(19),YY(20),YY(21),YY(22),YY(23),YY(24),YY(25),YY(26)
  Display : Display
  UCLC(1) Holdup of Component A (Liquid) in Stripper lb-mol : Gain
  UCLC(2) Holdup of Component B (Liquid) in Stripper lb-mol : Gain
  UCLC(3) Holdup of Component C (Liquid) in Stripper lb-mol : Gain
  UCLC(4) Holdup of Component D (Liquid) in Stripper lb-mol : Gain
  UCLC(5) Holdup of Component E (Liquid) in Stripper lb-mol : Gain
  UCLC(6) Holdup of Component F (Liquid) in Stripper lb-mol : Gain
  UCLC(7) Holdup of Component G (Liquid) in Stripper lb-mol : Gain
  UCLC(8) Holdup of Component H (Liquid) in Stripper lb-mol : Gain
  UCLC : Outport  VectorParamsAs1DForOutWhenUnconnected=off
  wires:
  UCLC(8) Holdup of Component H (Liquid) in Stripper lb-mol/1 -> Bus Creator/8
  UCLC(2) Holdup of Component B (Liquid) in Stripper lb-mol/1 -> Bus Creator/2
  UCLC(1) Holdup of Component A (Liquid) in Stripper lb-mol/1 -> Bus Creator/1
  Bus Creator/1 -> Display/1, UCLC/1
  UCLC(5) Holdup of Component E (Liquid) in Stripper lb-mol/1 -> Bus Creator/5
  UCLC(7) Holdup of Component G (Liquid) in Stripper lb-mol/1 -> Bus Creator/7
  UCLC(4) Holdup of Component D (Liquid) in Stripper lb-mol/1 -> Bus Creator/4
  UCLC(6) Holdup of Component F (Liquid) in Stripper lb-mol/1 -> Bus Creator/6
  UCLC(3) Holdup of Component C (Liquid) in Stripper lb-mol/1 -> Bus Creator/3
  YY(19:26)/1 -> Bus Selector/1
  Bus Selector/1 -> UCLC(1) Holdup of Component A (Liquid) in Stripper lb-mol/1  "<YY(19)>"
  Bus Selector/2 -> UCLC(2) Holdup of Component B (Liquid) in Stripper lb-mol/1  "<YY(20)>"
  Bus Selector/3 -> UCLC(3) Holdup of Component C (Liquid) in Stripper lb-mol/1  "<YY(21)>"
  Bus Selector/4 -> UCLC(4) Holdup of Component D (Liquid) in Stripper lb-mol/1  "<YY(22)>"
  Bus Selector/5 -> UCLC(5) Holdup of Component E (Liquid) in Stripper lb-mol/1  "<YY(23)>"
  Bus Selector/6 -> UCLC(6) Holdup of Component F (Liquid) in Stripper lb-mol/1  "<YY(24)>"
  Bus Selector/7 -> UCLC(7) Holdup of Component G (Liquid) in Stripper lb-mol/1  "<YY(25)>"
  Bus Selector/8 -> UCLC(8) Holdup of Component H (Liquid) in Stripper lb-mol/1  "<YY(26)>"

== system SP_Dynamic_17Okt_ExergyFlow/Stripper/Holdup of Components in Stripper/Liquid Component Fraction in Stripper ==
  UTLC : Inport
  UCLC : Inport  Port=2
  Bus Selector : BusSelector  OutputSignals=signal1,signal2,signal3,signal4,signal5,signal6,signal7,signal8
  Mux : Mux  Inputs=8
  XLC(1) : Product  Inputs=*/
  XLC(2) : Product  Inputs=*/
  XLC(3) : Product  Inputs=*/
  XLC(4) : Product  Inputs=*/
  XLC(5) : Product  Inputs=*/
  XLC(6) : Product  Inputs=*/
  XLC(7) : Product  Inputs=*/
  XLC(8) : Product  Inputs=*/
  XLC : Outport  VectorParamsAs1DForOutWhenUnconnected=off
  wires:
  XLC(3)/1 -> Mux/3  "XLC(3)"
  Bus Selector/2 -> XLC(2)/1  "<signal2>"
  Bus Selector/7 -> XLC(7)/1  "<signal7>"
  XLC(5)/1 -> Mux/5  "XLC(5)"
  XLC(7)/1 -> Mux/7  "XLC(7)"
  Bus Selector/3 -> XLC(3)/1  "<signal3>"
  UTLC/1 -> XLC(8)/2, XLC(7)/2, XLC(6)/2, XLC(5)/2, XLC(4)/2, XLC(3)/2, XLC(2)/2, XLC(1)/2
  Bus Selector/6 -> XLC(6)/1  "<signal6>"
  Bus Selector/5 -> XLC(5)/1  "<signal5>"
  XLC(2)/1 -> Mux/2  "XLC(2)"
  XLC(6)/1 -> Mux/6  "XLC(6)"
  Bus Selector/4 -> XLC(4)/1  "<signal4>"
  XLC(1)/1 -> Mux/1  "XLC(1)"
  XLC(8)/1 -> Mux/8  "XLC(8)"
  UCLC/1 -> Bus Selector/1
  XLC(4)/1 -> Mux/4  "XLC(4)"
  Mux/1 -> XLC/1
  Bus Selector/1 -> XLC(1)/1  "<signal1>"
  Bus Selector/8 -> XLC(8)/1  "<signal8>"

== system SP_Dynamic_17Okt_ExergyFlow/Stripper/Holdup of Components in Stripper/YP(19) ==
  FCM(1,12) : Inport
  FCM(1,13) : Inport  Port=2
  " " : Sum  Inputs=+-
  YP(19) : Integrator  InitialConditionSource=external
  "YY(19) " : Constant  Value=0.4306056376
  YY(19) : Outport  VectorParamsAs1DForOutWhenUnconnected=off
  wires:
  "YY(19) "/1 -> YP(19)/2
  FCM(1,13)/1 -> " "/2
  FCM(1,12)/1 -> " "/1
  " "/1 -> YP(19)/1
  YP(19)/1 -> YY(19)/1

== system SP_Dynamic_17Okt_ExergyFlow/Stripper/Holdup of Components in Stripper/YP(20) ==
  FCM(2,12) : Inport
  FCM(2,13) : Inport  Port=2
  " " : Sum  Inputs=+-
  YP(20) : Integrator  InitialConditionSource=external
  "YY(20) " : Constant  Value=7.9906200783E-3
  YY(20) : Outport  VectorParamsAs1DForOutWhenUnconnected=off
  wires:
  YP(20)/1 -> YY(20)/1
  FCM(2,12)/1 -> " "/1
  FCM(2,13)/1 -> " "/2
  "YY(20) "/1 -> YP(20)/2
  " "/1 -> YP(20)/1

== system SP_Dynamic_17Okt_ExergyFlow/Stripper/Holdup of Components in Stripper/YP(21) ==
  FCM(3,12) : Inport
  FCM(3,13) : Inport  Port=2
  " " : Sum  Inputs=+-
  YP(21) : Integrator  InitialConditionSource=external
  "YY(21) " : Constant  Value=0.9056036089
  YY(21) : Outport  VectorParamsAs1DForOutWhenUnconnected=off
  wires:
  YP(21)/1 -> YY(21)/1
  FCM(3,12)/1 -> " "/1
  FCM(3,13)/1 -> " "/2
  " "/1 -> YP(21)/1
  "YY(21) "/1 -> YP(21)/2

== system SP_Dynamic_17Okt_ExergyFlow/Stripper/Holdup of Components in Stripper/YP(22) ==
  FCM(4,12) : Inport
  FCM(4,13) : Inport  Port=2
  " " : Sum  Inputs=+-
  YP(22) : Integrator  InitialConditionSource=external
  "YY(22) " : Constant  Value=1.6054258216E-2
  "YY(22)  " : Outport  VectorParamsAs1DForOutWhenUnconnected=off
  wires:
  YP(22)/1 -> "YY(22)  "/1
  FCM(4,12)/1 -> " "/1
  FCM(4,13)/1 -> " "/2
  " "/1 -> YP(22)/1
  "YY(22) "/1 -> YP(22)/2

== system SP_Dynamic_17Okt_ExergyFlow/Stripper/Holdup of Components in Stripper/YP(23) ==
  FCM(5,12) : Inport
  FCM(5,13) : Inport  Port=2
  " " : Sum  Inputs=+-
  YP(23) : Integrator  InitialConditionSource=external
  "YY(23) " : Constant  Value=0.7509759687
  "YY(23)  " : Outport  VectorParamsAs1DForOutWhenUnconnected=off
  wires:
  YP(23)/1 -> "YY(23)  "/1
  FCM(5,12)/1 -> " "/1
  FCM(5,13)/1 -> " "/2
  " "/1 -> YP(23)/1
  "YY(23) "/1 -> YP(23)/2

== system SP_Dynamic_17Okt_ExergyFlow/Stripper/Holdup of Components in Stripper/YP(24) ==
  FCM(6,12) : Inport
  FCM(6,13) : Inport  Port=2
  " " : Sum  Inputs=+-
  YP(24) : Integrator  InitialConditionSource=external
  YY(24) : Constant  Value=8.8582855955E-2
  "YY(24)  " : Outport  VectorParamsAs1DForOutWhenUnconnected=off
  wires:
  YP(24)/1 -> "YY(24)  "/1
  FCM(6,12)/1 -> " "/1
  FCM(6,13)/1 -> " "/2
  " "/1 -> YP(24)/1
  YY(24)/1 -> YP(24)/2

== system SP_Dynamic_17Okt_ExergyFlow/Stripper/Holdup of Components in Stripper/YP(25) ==
  FCM(7,12) : Inport
  FCM(7,13) : Inport  Port=2
  " " : Sum  Inputs=+-
  YP(25) : Integrator  InitialConditionSource=external
  "YY(25) " : Constant  Value=48.27726193
  "YY(25)  " : Outport  VectorParamsAs1DForOutWhenUnconnected=off
  wires:
  YP(25)/1 -> "YY(25)  "/1
  FCM(7,12)/1 -> " "/1
  FCM(7,13)/1 -> " "/2
  " "/1 -> YP(25)/1
  "YY(25) "/1 -> YP(25)/2

== system SP_Dynamic_17Okt_ExergyFlow/Stripper/Holdup of Components in Stripper/YP(26) ==
  FCM(8,12) : Inport
  FCM(8,13) : Inport  Port=2
  " " : Sum  Inputs=+-
  YP(26) : Integrator  InitialConditionSource=external
  "YY(26) " : Constant  Value=39.38459028
  "YY(26)   " : Outport  VectorParamsAs1DForOutWhenUnconnected=off
  wires:
  YP(26)/1 -> "YY(26)   "/1
  FCM(8,12)/1 -> " "/1
  FCM(8,13)/1 -> " "/2
  " "/1 -> YP(26)/1
  "YY(26) "/1 -> YP(26)/2

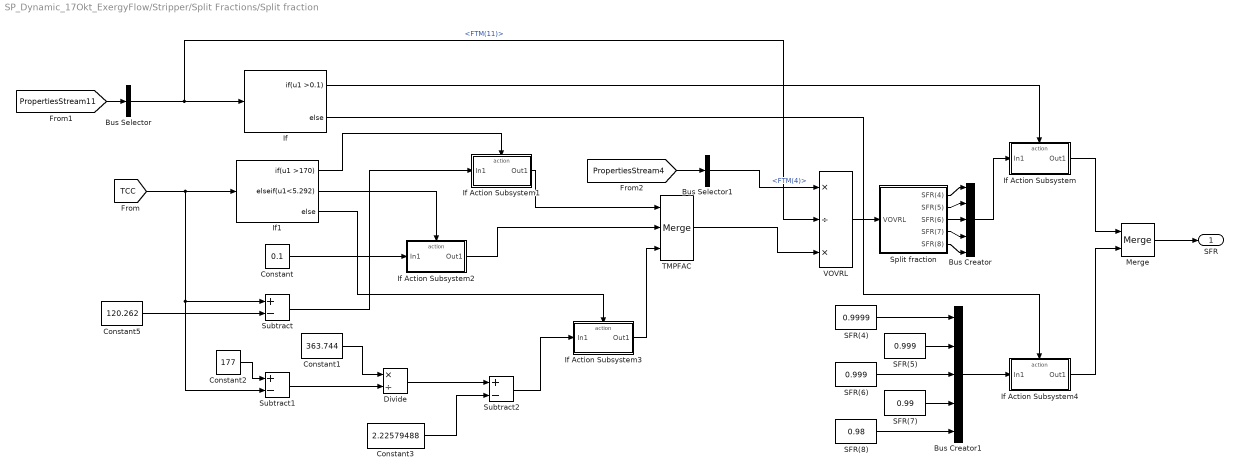
== system SP_Dynamic_17Okt_ExergyFlow/Stripper/Split Fractions/Split fraction ==
  Bus Creator : BusCreator  Inputs=5
  Bus Creator1 : BusCreator  Inputs=5
  Bus Selector : BusSelector  OutputSignals=signal1.FTM(11)
  Bus Selector1 : BusSelector  OutputSignals=FTM(4)
  Constant : Constant  Value=0.1
  Constant1 : Constant  Value=363.744
  Constant2 : Constant  Value=177
  Constant3 : Constant  Value=2.22579488
  Constant5 : Constant  Value=120.262
  Divide : Product  Inputs=*/
  If : If  IfExpression=u1 >0.1
  If Action Subsystem : Subsystem  TreatAsAtomicUnit=on
  If Action Subsystem1 : Subsystem  TreatAsAtomicUnit=on
  If Action Subsystem2 : Subsystem  TreatAsAtomicUnit=on
  If Action Subsystem3 : Subsystem  TreatAsAtomicUnit=on
  If Action Subsystem4 : Subsystem  TreatAsAtomicUnit=on
  If1 : If  IfExpression=u1 >170  ElseIfExpressions=u1<5.292
  Merge : Merge
  SFR(4) : Constant  Value=0.9999
  SFR(5) : Constant  Value=0.999
  SFR(6) : Constant  Value=0.999
  SFR(7) : Constant  Value=0.99
  SFR(8) : Constant  Value=0.98
  Split fraction : Subsystem
  Subtract : Sum  Inputs=+-
  Subtract1 : Sum  Inputs=+-
  Subtract2 : Sum  Inputs=+-
  "TMPFAC  " : Merge  Inputs=3
  VOVRL : Product  Inputs=*/*
  SFR : Outport  VectorParamsAs1DForOutWhenUnconnected=off
  wires:
  If/1 -> If Action Subsystem/Action
  Bus Selector/1 -> VOVRL/2, If/1  "<FTM(11)>"
  [TCC] -> If1/1, Subtract1/2, Subtract/1
  Constant5/1 -> Subtract/2
  Constant2/1 -> Subtract1/1
  Subtract1/1 -> Divide/2
  Constant1/1 -> Divide/1
  Divide/1 -> Subtract2/1
  Constant3/1 -> Subtract2/2
  If Action Subsystem1/1(Out1) -> "TMPFAC  "/1
  If Action Subsystem2/1(Out1) -> "TMPFAC  "/2
  If1/1 -> If Action Subsystem1/Action
  Subtract/1 -> If Action Subsystem1/1(In1)
  If1/2 -> If Action Subsystem2/Action
  Constant/1 -> If Action Subsystem2/1(In1)
  Subtract2/1 -> If Action Subsystem3/1(In1)
  If1/3 -> If Action Subsystem3/Action
  If Action Subsystem3/1(Out1) -> "TMPFAC  "/3
  Bus Selector1/1 -> VOVRL/1  "<FTM(4)>"
  "TMPFAC  "/1 -> VOVRL/3
  VOVRL/1 -> Split fraction/1(VOVRL)
  If/2 -> If Action Subsystem4/Action
  Split fraction/1(SFR(4)) -> Bus Creator/1
  Split fraction/2(SFR(5)) -> Bus Creator/2
  Split fraction/3(SFR(6)) -> Bus Creator/3
  Split fraction/4(SFR(7)) -> Bus Creator/4
  Split fraction/5(SFR(8)) -> Bus Creator/5
  Bus Creator/1 -> If Action Subsystem/1(In1)
  Bus Creator1/1 -> If Action Subsystem4/1(In1)
  SFR(4)/1 -> Bus Creator1/1
  SFR(5)/1 -> Bus Creator1/2
  SFR(6)/1 -> Bus Creator1/3
  SFR(7)/1 -> Bus Creator1/4
  SFR(8)/1 -> Bus Creator1/5
  If Action Subsystem4/1(Out1) -> Merge/2
  If Action Subsystem/1(Out1) -> Merge/1
  Merge/1 -> SFR/1
  [PropertiesStream11] -> Bus Selector/1
  [PropertiesStream4] -> Bus Selector1/1

== system SP_Dynamic_17Okt_ExergyFlow/Stripper/Stream 12/HST(12) Molar Enthalpy of Stream 12 MBtu//lb-mol ==
  ITY : Inport
  T : Inport  Port=2
  XST(I,I) : Inport  Port=3
  "Enthalpy of Stream " : mylib/Enthalpy of Stream   SystemSampleTime=-1  Latency=0  AutoFrameSizeCalculation=off
  "H " : Outport  VectorParamsAs1DForOutWhenUnconnected=off
  wires:
  ITY/1 -> "Enthalpy of Stream "/1
  T/1 -> "Enthalpy of Stream "/2
  XST(I,I)/1 -> "Enthalpy of Stream "/3
  "Enthalpy of Stream "/1 -> "H "/1

== system SP_Dynamic_17Okt_ExergyFlow/Stripper/Stream 13/HST(13) Molar Enthalpy of Stream 13 MBtu//lb-mol ==
  ITY : Inport
  T : Inport  Port=2
  XST(I,I) : Inport  Port=3
  "Enthalpy of Stream " : mylib/Enthalpy of Stream   SystemSampleTime=-1  Latency=0  AutoFrameSizeCalculation=off
  "H " : Outport  VectorParamsAs1DForOutWhenUnconnected=off
  wires:
  ITY/1 -> "Enthalpy of Stream "/1
  T/1 -> "Enthalpy of Stream "/2
  XST(I,I)/1 -> "Enthalpy of Stream "/3
  "Enthalpy of Stream "/1 -> "H "/1

== system SP_Dynamic_17Okt_ExergyFlow/Stripper/Stream 5/HST(5) Molar Enthalpy of Stream 5 MBtu//lb-mol ==
  ITY : Inport
  TST(5) : Inport  Port=2
  XST(I,5) : Inport  Port=3
  "Enthalpy of Stream " : mylib/Enthalpy of Stream   SystemSampleTime=-1  Latency=0  AutoFrameSizeCalculation=off
  "H " : Outport  PortDimensions=1  VectorParamsAs1DForOutWhenUnconnected=off
  wires:
  ITY/1 -> "Enthalpy of Stream "/1
  TST(5)/1 -> "Enthalpy of Stream "/2
  XST(I,5)/1 -> "Enthalpy of Stream "/3
  "Enthalpy of Stream "/1 -> "H "/1

== system SP_Dynamic_17Okt_ExergyFlow/Stripper/Volume of Stripper/DLC Molar Density of Liquids in Stripper lb-mol//ft³     ==
  XLC : Inport
  TCC : Inport  Port=2
  "DLC Molar Density of Liquids in Stripper lb-mol/ft³ " : Subsystem
  "DLC " : Outport  VectorParamsAs1DForOutWhenUnconnected=off
  wires:
  "DLC Molar Density of Liquids in Stripper lb-mol/ft³ "/1("R ") -> "DLC "/1
  TCC/1 -> "DLC Molar Density of Liquids in Stripper lb-mol/ft³ "/2(T)
  XLC/1 -> "DLC Molar Density of Liquids in Stripper lb-mol/ft³ "/1(X)

== system SP_Dynamic_17Okt_ExergyFlow/Subsystem/Braatz/  ==
  XMEAS : Inport
  Bus Selector : BusSelector  OutputSignals=signal1.XMEAS(2),signal8.XMEAS(26)
  CONTROL 1 : Subsystem
  CONTROL 14 : Subsystem
  XMV(1) : Outport  VectorParamsAs1DForOutWhenUnconnected=off
  wires:
  CONTROL 1/1(XMV(1)) -> XMV(1)/1
  CONTROL 14/1(SETPT(1)) -> CONTROL 1/2(SETPT(1))
  XMEAS/1 -> Bus Selector/1
  Bus Selector/1 -> CONTROL 1/1(XMEAS(2))  "<XMEAS(2)>"
  Bus Selector/2 -> CONTROL 14/1(XMEAS(26))  "<XMEAS(26)>"

== system SP_Dynamic_17Okt_ExergyFlow/Subsystem/Braatz/ 1 ==
  XMEAS : Inport
  Bus Selector : BusSelector  OutputSignals=signal1.XMEAS(3),signal8.XMEAS(27)
  CONTROL 15 : Subsystem
  CONTROL 2 : Subsystem
  XMV(2) : Outport  VectorParamsAs1DForOutWhenUnconnected=off
  wires:
  CONTROL 2/1(XMV(2)) -> XMV(2)/1
  CONTROL 15/1(SETPT(2)) -> CONTROL 2/2(SETPT(2))
  XMEAS/1 -> Bus Selector/1
  Bus Selector/1 -> CONTROL 2/1(XMEAS(2))  "<XMEAS(3)>"
  Bus Selector/2 -> CONTROL 15/1(XMEAS(27))  "<XMEAS(27)>"

== system SP_Dynamic_17Okt_ExergyFlow/Subsystem/Braatz/ 10 ==
  XMEAS : Inport
  Bus Selector : BusSelector  OutputSignals=signal9.XMEAS(30)
  CONTROL 19 : Subsystem
  CONTROL 6 : Subsystem
  XMV(6) : Outport  VectorParamsAs1DForOutWhenUnconnected=off
  wires:
  CONTROL 6/1(XMV(6)) -> XMV(6)/1
  CONTROL 19/1(SETPT(6)) -> CONTROL 6/1(SETPT(6))
  XMEAS/1 -> CONTROL 6/2(XMEAS), Bus Selector/1
  Bus Selector/1 -> CONTROL 19/1(XMEAS(30))  "<XMEAS(30)>"

== system SP_Dynamic_17Okt_ExergyFlow/Subsystem/Braatz/ 2 ==
  XMEAS : Inport
  Bus Selector : BusSelector  OutputSignals=signal1.XMEAS(1),signal8.XMEAS(23)
  CONTROL 13 : Subsystem
  CONTROL 3 : Subsystem
  Scope : Scope
  XMV(3) : Outport  VectorParamsAs1DForOutWhenUnconnected=off
  wires:
  CONTROL 3/1(XMV(3)) -> XMV(3)/1
  CONTROL 13/1(SETPT(3)) -> Scope/1, CONTROL 3/2(SETPT(3))
  XMEAS/1 -> Bus Selector/1
  Bus Selector/1 -> CONTROL 3/1(XMEAS(1))  "<XMEAS(1)>"
  Bus Selector/2 -> CONTROL 13/1(XMEAS(23))  "<XMEAS(23)>"

== system SP_Dynamic_17Okt_ExergyFlow/Subsystem/Braatz/ 3 ==
  XMEAS : Inport
  Bus Selector : BusSelector  OutputSignals=signal1.XMEAS(4),signal2.XMEAS(8)
  CONTROL 17 : Subsystem
  CONTROL 4 : Subsystem
  XMV(4) : Outport  VectorParamsAs1DForOutWhenUnconnected=off
  wires:
  CONTROL 4/1(XMV(4)) -> XMV(4)/1
  CONTROL 17/1(SETPT(4)) -> CONTROL 4/2(SETPT(4))
  XMEAS/1 -> Bus Selector/1
  Bus Selector/1 -> CONTROL 4/1(XMEAS(4))  "<XMEAS(4)>"
  Bus Selector/2 -> CONTROL 17/1(XMEAS(8))  "<XMEAS(8)>"
